simulink model "line_algo"  (R2017a)
settings: Solver=VariableStepAuto  StartTime=0.0  StopTime=10.0  RelTol=1e-3
undefined symbols (not defined in the file): Line_Scan_Value
settings Model: Creator=trey  LastModifiedBy=trey

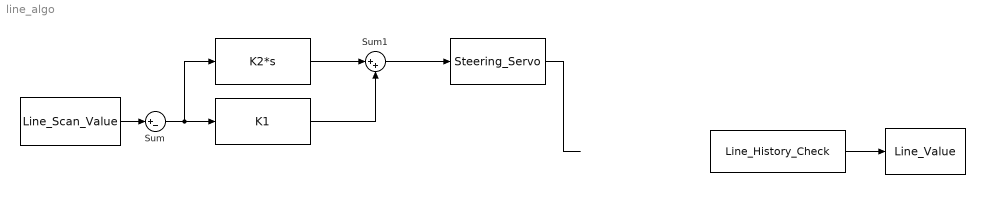
== system line_algo ==
  " " : ToWorkspace  VariableName=Line_Value  SaveFormat=Timeseries  SampleTime=-1
  "   " : Constant  Value=Line_Scan_Value
  "    " : S-Function  FunctionName=K1  SFunctionDeploymentMode=off  EnableBusSupport=off
  "          " : S-Function  FunctionName=K2*s  SFunctionDeploymentMode=off  EnableBusSupport=off
  "           " : S-Function  FunctionName=Steering_Servo  SFunctionDeploymentMode=off  EnableBusSupport=off
  "             " : S-Function  FunctionName=Line_History_Check  SFunctionDeploymentMode=off  EnableBusSupport=off
  Sum : Sum  Inputs=|+-
  Sum1 : Sum  Inputs=|++
  wires:
  "           "/1 -> ?
  "             "/1 -> " "/1
  ? -> "             "/1
  "   "/1 -> Sum/1
  Sum/1 -> "          "/1, "    "/1
  "          "/1 -> Sum1/1
  "    "/1 -> Sum1/2
  Sum1/1 -> "           "/1
